simulink model "MPC_Controllers_P1"  (R2020b)
settings: Solver=VariableStepAuto  StartTime=0.0  StopTime=0.3  RelTol=1e-3
values from neighbouring files (symbols this model uses):
  Bm = 0.05    [IniVar.m]
  Jm = 0.001    [IniVar.m]
  Km = 0.5    [IniVar.m]
  Nm = 2    [IniVar.m]
libraries: MPC_Controllers x1
settings Model: Creator=snopv  LastModifiedBy=snopv

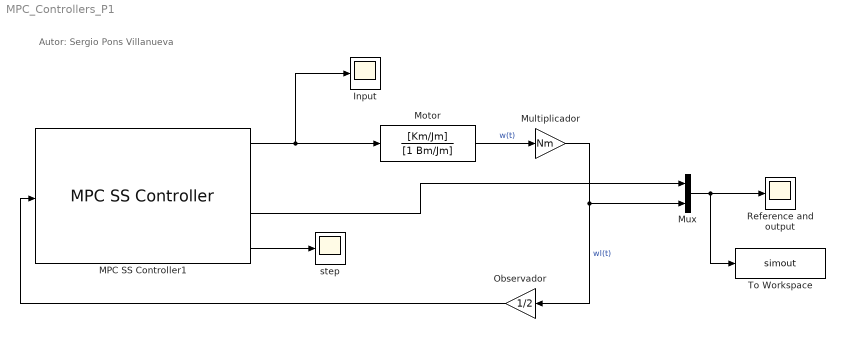
== system MPC_Controllers_P1 ==
  note: Autor: Sergio Pons Villanueva
  Input : Scope
  MPC SS Controller1 : MPC_Controllers/MPC SS Controller
  Motor : TransferFcn  Numerator=[Km/Jm]  Denominator=[1 Bm/Jm]
  Multiplicador : Gain  Gain=Nm
  Mux : Mux  Inputs=2
  Observador : Gain  Gain=1/2
  Reference and output : Scope
  To Workspace : ToWorkspace  VariableName=simout  SaveFormat=Timeseries  SampleTime=-1
  step : Scope
  wires:
  Observador/1 -> MPC SS Controller1/1
  MPC SS Controller1/3 -> Mux/1
  Motor/1 -> Multiplicador/1  "w(t)"
  Mux/1 -> To Workspace/1, Reference and output/1
  MPC SS Controller1/1 -> Input/1, Motor/1
  Multiplicador/1 -> Mux/2, Observador/1  "wl(t)"
  MPC SS Controller1/4 -> step/1
